simulink model "furnace_emul_v12"  (Simulink 5.0)
settings: Solver=FixedStepDiscrete  StartTime=0.0  StopTime=9000  RelTol=1e-3
values from neighbouring files (symbols this model uses):
  A_amb = pi*(D_e+2*d_ins)*L    (= 0.0498884492)    [tube_ini.m]
  A_e = pi*D_e*L    (= 0.0247557292)    [tube_ini.m]
  A_pi = pi*D_pi*L    (= 0.017592904)    [tube_ini.m]
  A_po = pi*D_po*L    (= 0.0184725492)    [tube_ini.m]
  A_w = pi/4*D_w^2*n_sl    (= 0.0628318)    [tube_ini.m]
  A_wc = pi*D_w*Li    (= 0.01256636)    [tube_ini.m]
  D_pi = D_w+2*DX_R    (= 0.28)    [tube_ini.m]
  D_w = 0.2    [tube_ini.m]
  elem_tmax = 1250    [tube_ini.m]
  F_A_e = lam_p_bct*F_A_e+lam_p_bcb*F_A_e([n:-1:1])    [tube_ini.m]
  F_A_ew = e_ew*A_ew./((1/ei-1)+(1/eo-1)*D_pi/D_w+1./(toeplitz(F1*Li)))    [tube_ini.m]
  F_A_p = lam_p_bct*F_A_p+lam_p_bcb*F_A_p([n:-1:1])    [tube_ini.m]
  F_A_pe = A_ep./((1/ei-1)+(1/eo-1)*D_po/D_e+1./(toeplitz(F1*Li)))    [tube_ini.m]
  F_A_pw = A_pw./((1/ei-1)+(1/eo-1)*D_pi/D_w+1./(toeplitz(F1*Li)))    [tube_ini.m]
  f_amb_ped = 1    [tube_ini.m]
  f_amb_top = .3    (= 0.3)    [tube_ini.m]
  Fb_A_ew = e_ew*Aib./((1/ei-1)+(1/eo-1)*Aib/A+1./(F4*Li))    [tube_ini.m]
  Fb_A_pw = Aib./((1/ei-1)+(1/eo-1)*Aib/A+1./(F4*Li))    [tube_ini.m]
  Fs_e = e_ew*A_e./((1/eo-1)+(1/eo-1)+1./(toeplitz(F5*Li)))    [tube_ini.m]
  Fs_p = A_pi./((1/eo-1)+(1/eo-1)+1./(toeplitz(F5*Li)))    [tube_ini.m]
  gww_bot = ones(N_w,1)*SW    [tube_ini.m]
  gww_top = gww_bot    [tube_ini.m]
  h_amb = 1    [tube_ini.m]
  h_gas = 2    [tube_ini.m]
  H_Z = zeros(n,5)    [tube_ini.m]
  k_adj_ped = 0.6    [tube_ini.m]
  k_adj_top = 0.5    [tube_ini.m]
  L = 0.2    [M_Hist040407.m]    (also in exp303.m = 500:499+ly; tube_ini.m = 0.02)
  lam_p_bcb = 1    [tube_ini.m]
  lam_p_bct = .4    (= 0.4)    [tube_ini.m]
  Li = dx_w    (= 0.02)    [tube_ini.m]
  m_e = rho_e*V_e    (= 0.6312710946)    [tube_ini.m]
  m_p = V_p*rho_p    (= 0.30294980688)    [tube_ini.m]
  m_ped = V_ped*rho_p    (= 1.5079632)    [tube_ini.m]
  m_top = rho_p*V_top    (= 1.5079632)    [tube_ini.m]
  m_w = rho_w*V_w    (= 0.146398094)    [tube_ini.m]
  mcp_adj_ped = 0.36    [tube_ini.m]
  mcp_adj_top = 0.25    [tube_ini.m]
  n = N_w+N_top+N_ped    [tube_ini.m]
  N_ped = round(DX_P/Li)    [tube_ini.m]
  N_top = n-N_w-N_p    [s_tubew.m]    (also in tube_ini.m = round(DX_T/Li))
  N_w = 100/n_sl    (= 50)    [tube_ini.m]
  pow_pm = pow_pml*pi*D_e*n*L/(d_e+d_g)    [tube_ini.m]
  pr_gas = 0.2    [tube_ini.m]
  PRG = 0*SPE; for ii=1:length(profile_loc); PRG(ii,profile_loc(ii))=1;end    [tube_ini.m]
  profile_loc = [N_top,h_zones(1)+round(h_zones(2)/2),   sum(h_zones(1:2))+round(h_zones(3)/2),sum(h_zones(1:3))+round(h_zones(4)/2),   n-N_ped]    [tube_ini.m]
  PRT = PRT'    [tube_ini.m]
  PRW = PRW'    [tube_ini.m]
  SPE = SPE'    [tube_ini.m]
  spike_loc = [round(h_zones(1)/2),h_zones(1)+round(h_zones(2)/2),   sum(h_zones(1:2))+round(h_zones(3)/2),sum(h_zones(1:3))+round(h_zones(4)/2),   sum(h_zones(1:4))+round(h_zones(5)/2)]    [tube_ini.m]
  SPT = SPT'    [tube_ini.m]
  T_0 = T_01*ones(n,1)    [tube_ini.m]
  T_a0 = T_a01*ones(n,1)    [tube_ini.m]
  T_amb = 25    [tube_ini.m]
  T_w0 = T_amb*ones(N_w,1)    [tube_ini.m]
  T_w0_ped = T_amb*ones(N_ped,1)    [tube_ini.m]
  T_w0_top = T_01*ones(N_top,1)    [tube_ini.m]
  Tsa = .5    (= 0.5)    [tube_ini.m]
  tube_tmax = 1200    [tube_ini.m]
  V_a = pi/4*D_pi^2*L    (= 0.00123150328)    [tube_ini.m]
undefined symbols (not defined in the file or in its folder): N, s_tubew
libraries: simulink3 x19, simulink x2
(part 1 of 2)
settings Model: LastModifiedBy="Kostas  Tsakalis"  BlockReductionOpt=off  BooleanDataType=off  RTWOptions="-aEnforceIntegerDowncast=1 -aExtMode=0 -aFoldNonRolledExpr=1 -aForceParamTrailComments=0 -aGenerateComments=1 -aIgnoreCustomStorageClasses=0 -aIncHierarchyInIds=0 -aInlineInvariantSignals=0 -aLocalBlockOutputs=1 -aLogVarNameModifier=\"rt_\" -aRTWVerbose=1 -aRollThreshold=5 -aShowEliminatedStatements=1"

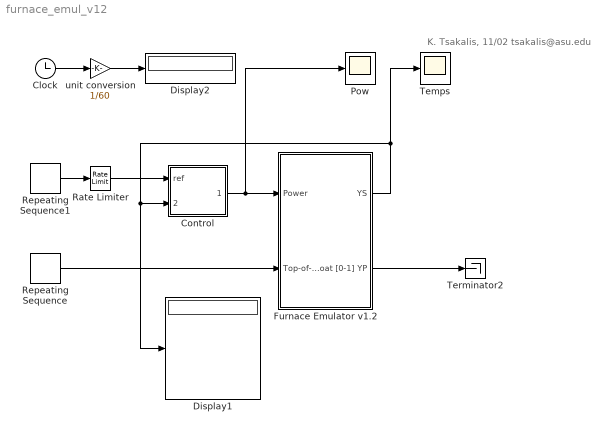
== system furnace_emul_v12 ==
  note: K. Tsakalis, 11/02
      | tsakalis@asu.edu
  Clock : Clock
      settings: Decimation=10
  Control : Subsystem
      mask init:
      | Tsa=0.5;
  Display1 : Display
      settings: Format=short_e
  Display2 : Display
      settings: Format=short_e
  Furnace Emulator v1.2 : Subsystem
      mask init:
      | tube_ini;
  Pow : Scope
      settings: TimeRange=6000  YMin=0  YMax=1
  Rate Limiter : RateLimiter  RisingSlewLimit=250/60  FallingSlewLimit=-200/60
  Repeating Sequence : simulink/Sources/Repeating Sequence  rep_seq_t="[0,  20,  22,  130,  132,  150]*60"  rep_seq_y="[1,  1,  0,  0,  1,  1]"
  Repeating Sequence1 : simulink/Sources/Repeating Sequence  rep_seq_t="[0,  35,  35.0001,  70,   70.0001  150 ]*60"  rep_seq_y="[0,  0,  300,  300,  0,  0]+600"
  Temps : Scope
      settings: TimeRange=6000  YMin=500  YMax=1000
  Terminator2 : Terminator
  unit conversion : Gain  Gain=1/60  SaturateOnIntegerOverflow=on
  wires:
  Furnace Emulator v1.2/1(YS) -> Temps/1, Control/2(meas), Display1/1
  Furnace Emulator v1.2/2(YP) -> Terminator2/1
  Clock/1 -> unit conversion/1
  Repeating Sequence1/1 -> Rate Limiter/1
  Control/1(Out1) -> Furnace Emulator v1.2/1(Power), Pow/1
  Rate Limiter/1 -> Control/1(ref)
  Repeating Sequence/1 -> Furnace Emulator v1.2/2(Top-of-boat [0-1])
  unit conversion/1 -> Display2/1

== system furnace_emul_v12/Control ==
  ref : Inport
  meas : Inport  Port=2
  "AW-PID " : Subsystem  mask(Anti-windup PID ){@1=[.005, 50, 10], @2=1, @3=0, @4=Tsa, @5=[1 0]}
      mask prompts: @1 "Gain kp - Integral time ki - Derivative time kd"; @2 "Pseudo-derivative filter time constant"; @3 "Error lowpass filter Time constant"; @4 "Sampling Time"; @5 "Saturation Limits [umax umin]"
      mask help: Discrete PID with Anti-windup and with lowpass filter
      mask init:
      | kp=@1(1);ki=@1(2);kd=@1(3);SAM=@2;TF=@3;DT=@4;umax=@5(1);umin=@5(2);
      mask Display: disp('AW-PID+filter')
  AW-PID 1 : Subsystem  mask(Anti-windup PID ){@1=[.005, 50, 10], @2=1, @3=0, @4=Tsa, @5=[1 0]}
      mask prompts: @1 "Gain kp - Integral time ki - Derivative time kd"; @2 "Pseudo-derivative filter time constant"; @3 "Error lowpass filter Time constant"; @4 "Sampling Time"; @5 "Saturation Limits [umax umin]"
      mask help: Discrete PID with Anti-windup and with lowpass filter
      mask init:
      | kp=@1(1);ki=@1(2);kd=@1(3);SAM=@2;TF=@3;DT=@4;umax=@5(1);umin=@5(2);
      mask Display: disp('AW-PID+filter')
  AW-PID 2 : Subsystem  mask(Anti-windup PID ){@1=[.005, 50, 10], @2=1, @3=0, @4=Tsa, @5=[1 0]}
      mask prompts: @1 "Gain kp - Integral time ki - Derivative time kd"; @2 "Pseudo-derivative filter time constant"; @3 "Error lowpass filter Time constant"; @4 "Sampling Time"; @5 "Saturation Limits [umax umin]"
      mask help: Discrete PID with Anti-windup and with lowpass filter
      mask init:
      | kp=@1(1);ki=@1(2);kd=@1(3);SAM=@2;TF=@3;DT=@4;umax=@5(1);umin=@5(2);
      mask Display: disp('AW-PID+filter')
  AW-PID 3 : Subsystem  mask(Anti-windup PID ){@1=[.005, 50, 10], @2=1, @3=0, @4=Tsa, @5=[1 0]}
      mask prompts: @1 "Gain kp - Integral time ki - Derivative time kd"; @2 "Pseudo-derivative filter time constant"; @3 "Error lowpass filter Time constant"; @4 "Sampling Time"; @5 "Saturation Limits [umax umin]"
      mask help: Discrete PID with Anti-windup and with lowpass filter
      mask init:
      | kp=@1(1);ki=@1(2);kd=@1(3);SAM=@2;TF=@3;DT=@4;umax=@5(1);umin=@5(2);
      mask Display: disp('AW-PID+filter')
  AW-PID 4 : Subsystem  mask(Anti-windup PID ){@1=[.005, 50, 10], @2=1, @3=0, @4=Tsa, @5=[1 0]}
      mask prompts: @1 "Gain kp - Integral time ki - Derivative time kd"; @2 "Pseudo-derivative filter time constant"; @3 "Error lowpass filter Time constant"; @4 "Sampling Time"; @5 "Saturation Limits [umax umin]"
      mask help: Discrete PID with Anti-windup and with lowpass filter
      mask init:
      | kp=@1(1);ki=@1(2);kd=@1(3);SAM=@2;TF=@3;DT=@4;umax=@5(1);umin=@5(2);
      mask Display: disp('AW-PID+filter')
  Mux1 : Mux  Inputs=5
  Selector1 : Selector  Elements=2  InputPortWidth=5
  Selector2 : Selector  Elements=3  InputPortWidth=5
  Selector3 : Selector  Elements=4  InputPortWidth=5
  Selector4 : Selector  Elements=5  InputPortWidth=5
  Selector5 : Selector  InputPortWidth=5
  Out1 : Outport
  wires:
  ref/1 -> "AW-PID "/1(Set point), AW-PID 1/1(Set point), AW-PID 2/1(Set point), AW-PID 3/1(Set point), AW-PID 4/1(Set point)
  Mux1/1 -> Out1/1
  meas/1 -> Selector5/1, Selector1/1, Selector2/1, Selector3/1, Selector4/1
  Selector5/1 -> "AW-PID "/2(System Output)
  Selector4/1 -> AW-PID 4/2(System Output)
  Selector3/1 -> AW-PID 3/2(System Output)
  Selector2/1 -> AW-PID 2/2(System Output)
  Selector1/1 -> AW-PID 1/2(System Output)
  AW-PID 2/1(Input to system) -> Mux1/3
  "AW-PID "/1(Input to system) -> Mux1/1
  AW-PID 1/1(Input to system) -> Mux1/2
  AW-PID 3/1(Input to system) -> Mux1/4
  AW-PID 4/1(Input to system) -> Mux1/5

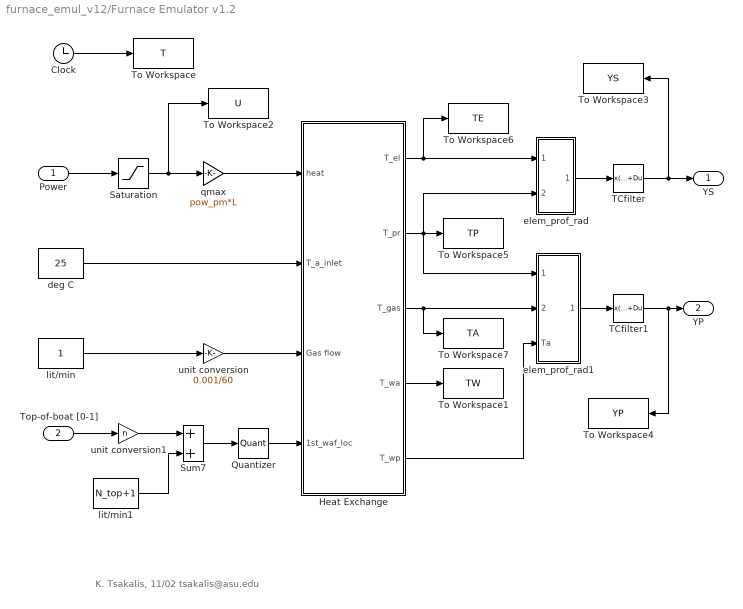
== system furnace_emul_v12/Furnace Emulator v1.2 ==
  note: K. Tsakalis, 11/02
      | tsakalis@asu.edu
  Power : Inport
  Top-of-boat [0-1] : Inport  Port=2
  Clock : Clock
      settings: Decimation=10
  Heat Exchange : Subsystem
  Quantizer : Quantizer  QuantizationInterval=1
  Saturation : Saturate  UpperLimit=1  LowerLimit=0
  Sum7 : Sum  Inputs=2  SaturateOnIntegerOverflow=on  InputSameDT=on
  TCfilter : DiscreteStateSpace  A=eye(5,5)-eye(5,5)*0.1*Tsa  B=eye(5,5)*0.1*Tsa  C=eye(5,5)  D=zeros(5,5)  X0=T_0(spike_loc)  SampleTime=Tsa
  TCfilter1 : DiscreteStateSpace  A=eye(5,5)-eye(5,5)*0.1*Tsa  B=eye(5,5)*0.1*Tsa  C=eye(5,5)  D=zeros(5,5)  X0=(T_0(profile_loc)*0.8+T_a0(profile_loc)*0.2)  SampleTime=Tsa
  To Workspace : ToWorkspace  VariableName=T  SampleTime=Tsa  SaveFormat=Array
      settings: Decimation=decim
  To Workspace1 : ToWorkspace  VariableName=TW  SampleTime=Tsa  SaveFormat=Array
      settings: Decimation=decim
  To Workspace2 : ToWorkspace  VariableName=U  SampleTime=Tsa  SaveFormat=Array
      settings: Decimation=decim
  To Workspace3 : ToWorkspace  VariableName=YS  SampleTime=Tsa  SaveFormat=Array
      settings: Decimation=decim
  To Workspace4 : ToWorkspace  VariableName=YP  SampleTime=Tsa  SaveFormat=Array
      settings: Decimation=decim
  To Workspace5 : ToWorkspace  VariableName=TP  SampleTime=Tsa  SaveFormat=Array
      settings: Decimation=decim
  To Workspace6 : ToWorkspace  VariableName=TE  SampleTime=Tsa  SaveFormat=Array
      settings: Decimation=decim
  To Workspace7 : ToWorkspace  VariableName=TA  SampleTime=Tsa  SaveFormat=Array
      settings: Decimation=decim
  deg C : Constant  Value=25
  elem_prof_rad : Subsystem
  elem_prof_rad1 : Subsystem
  lit/min : Constant
  lit/min1 : Constant  Value=N_top+1
  qmax : Gain  Gain=pow_pm*L  SaturateOnIntegerOverflow=on
  unit conversion : Gain  Gain=0.001/60  SaturateOnIntegerOverflow=on
  unit conversion1 : Gain  Gain=n  SaturateOnIntegerOverflow=on
  YS : Outport
  YP : Outport  Port=2
  wires:
  unit conversion/1 -> Heat Exchange/3(Gas flow)
  Power/1 -> Saturation/1
  Saturation/1 -> qmax/1, To Workspace2/1
  deg C/1 -> Heat Exchange/2(T_a_inlet)
  qmax/1 -> Heat Exchange/1(heat)
  Heat Exchange/1(T_el) -> To Workspace6/1, elem_prof_rad/1(Tel)
  Heat Exchange/2(T_pr) -> To Workspace5/1, elem_prof_rad/2(Ttu), elem_prof_rad1/1(Ttu)
  Heat Exchange/4(T_wa) -> To Workspace1/1
  Heat Exchange/3(T_gas) -> To Workspace7/1, elem_prof_rad1/2(Twa)
  elem_prof_rad/1(Tav) -> TCfilter/1
  elem_prof_rad1/1(Tav) -> TCfilter1/1
  TCfilter/1 -> YS/1, To Workspace3/1
  TCfilter1/1 -> YP/1, To Workspace4/1
  Clock/1 -> To Workspace/1
  Heat Exchange/5(T_wp) -> elem_prof_rad1/3(Ta)
  Top-of-boat [0-1]/1 -> unit conversion1/1
  lit/min/1 -> unit conversion/1
  Quantizer/1 -> Heat Exchange/4(1st_waf_loc)
  Sum7/1 -> Quantizer/1
  unit conversion1/1 -> Sum7/1
  lit/min1/1 -> Sum7/2

== system furnace_emul_v12/Control/AW-PID  ==
  Set point : Inport
  System Output : Inport  Port=2
  Constant : Constant  Value=0
  Dis. Transfer Fcn1 : DiscreteTransferFcn  Numerator=[DT/SAM]  Denominator=[1 -1+DT/SAM]  SampleTime=DT
  Low-pass filter : DiscreteTransferFcn  Numerator="[DT/(TF+DT),  0]"  Denominator="[1,  -TF/(TF+DT)]"  SampleTime=DT
  P+I+D : Sum  Inputs=++++-  SaturateOnIntegerOverflow=on  InputSameDT=on
  Proportional : Gain  Gain=kp  SaturateOnIntegerOverflow=on
  Proportional3 : Gain  Gain=kp*kd/SAM  SaturateOnIntegerOverflow=on
  Saturation : Saturate  UpperLimit=umax  LowerLimit=umin
  error : Sum  Inputs=+-  SaturateOnIntegerOverflow=on  InputSameDT=on
  gain : Gain  Gain=DT*kp/ki  SaturateOnIntegerOverflow=on
  integrator2 : Subsystem  mask(Anti windup intgrator){@1=umax, @2=umin, @3=DT}
      mask prompts: @1 "umax"; @2 "umin"; @3 "sampling time"
      mask help: Integral with anti-windup
      mask init:
      | umax=@1 ; umin =@2 ;DT=@3;
      mask Display: disp('DT-I-AW')
  Input to system : Outport  InitialOutput=0
  wires:
  integrator2/1(out_1) -> P+I+D/1
  error/1 -> Low-pass filter/1
  Set point/1 -> error/1
  System Output/1 -> error/2
  Proportional3/1 -> Dis. Transfer Fcn1/1, P+I+D/4
  Low-pass filter/1 -> Proportional/1, Proportional3/1, gain/1
  Dis. Transfer Fcn1/1 -> P+I+D/5
  Proportional/1 -> P+I+D/3
  gain/1 -> integrator2/1(in_1)
  P+I+D/1 -> Saturation/1
  Saturation/1 -> Input to system/1
  Constant/1 -> P+I+D/2

== system furnace_emul_v12/Control/AW-PID 1 ==
  Set point : Inport
  System Output : Inport  Port=2
  Constant : Constant  Value=0
  Dis. Transfer Fcn1 : DiscreteTransferFcn  Numerator=[DT/SAM]  Denominator=[1 -1+DT/SAM]  SampleTime=DT
  Low-pass filter : DiscreteTransferFcn  Numerator="[DT/(TF+DT),  0]"  Denominator="[1,  -TF/(TF+DT)]"  SampleTime=DT
  P+I+D : Sum  Inputs=++++-  SaturateOnIntegerOverflow=on  InputSameDT=on
  Proportional : Gain  Gain=kp  SaturateOnIntegerOverflow=on
  Proportional3 : Gain  Gain=kp*kd/SAM  SaturateOnIntegerOverflow=on
  Saturation : Saturate  UpperLimit=umax  LowerLimit=umin
  error : Sum  Inputs=+-  SaturateOnIntegerOverflow=on  InputSameDT=on
  gain : Gain  Gain=DT*kp/ki  SaturateOnIntegerOverflow=on
  integrator2 : Subsystem  mask(Anti windup intgrator){@1=umax, @2=umin, @3=DT}
      mask prompts: @1 "umax"; @2 "umin"; @3 "sampling time"
      mask help: Integral with anti-windup
      mask init:
      | umax=@1 ; umin =@2 ;DT=@3;
      mask Display: disp('DT-I-AW')
  Input to system : Outport  InitialOutput=0
  wires:
  Constant/1 -> P+I+D/2
  Saturation/1 -> Input to system/1
  P+I+D/1 -> Saturation/1
  gain/1 -> integrator2/1(in_1)
  Proportional/1 -> P+I+D/3
  Dis. Transfer Fcn1/1 -> P+I+D/5
  Low-pass filter/1 -> gain/1, Proportional3/1, Proportional/1
  Proportional3/1 -> P+I+D/4, Dis. Transfer Fcn1/1
  System Output/1 -> error/2
  Set point/1 -> error/1
  error/1 -> Low-pass filter/1
  integrator2/1(out_1) -> P+I+D/1

== system furnace_emul_v12/Control/AW-PID 2 ==
  Set point : Inport
  System Output : Inport  Port=2
  Constant : Constant  Value=0
  Dis. Transfer Fcn1 : DiscreteTransferFcn  Numerator=[DT/SAM]  Denominator=[1 -1+DT/SAM]  SampleTime=DT
  Low-pass filter : DiscreteTransferFcn  Numerator="[DT/(TF+DT),  0]"  Denominator="[1,  -TF/(TF+DT)]"  SampleTime=DT
  P+I+D : Sum  Inputs=++++-  SaturateOnIntegerOverflow=on  InputSameDT=on
  Proportional : Gain  Gain=kp  SaturateOnIntegerOverflow=on
  Proportional3 : Gain  Gain=kp*kd/SAM  SaturateOnIntegerOverflow=on
  Saturation : Saturate  UpperLimit=umax  LowerLimit=umin
  error : Sum  Inputs=+-  SaturateOnIntegerOverflow=on  InputSameDT=on
  gain : Gain  Gain=DT*kp/ki  SaturateOnIntegerOverflow=on
  integrator2 : Subsystem  mask(Anti windup intgrator){@1=umax, @2=umin, @3=DT}
      mask prompts: @1 "umax"; @2 "umin"; @3 "sampling time"
      mask help: Integral with anti-windup
      mask init:
      | umax=@1 ; umin =@2 ;DT=@3;
      mask Display: disp('DT-I-AW')
  Input to system : Outport  InitialOutput=0
  wires:
  integrator2/1(out_1) -> P+I+D/1
  error/1 -> Low-pass filter/1
  Set point/1 -> error/1
  System Output/1 -> error/2
  Proportional3/1 -> Dis. Transfer Fcn1/1, P+I+D/4
  Low-pass filter/1 -> Proportional/1, Proportional3/1, gain/1
  Dis. Transfer Fcn1/1 -> P+I+D/5
  Proportional/1 -> P+I+D/3
  gain/1 -> integrator2/1(in_1)
  P+I+D/1 -> Saturation/1
  Saturation/1 -> Input to system/1
  Constant/1 -> P+I+D/2

== system furnace_emul_v12/Control/AW-PID 3 ==
  Set point : Inport
  System Output : Inport  Port=2
  Constant : Constant  Value=0
  Dis. Transfer Fcn1 : DiscreteTransferFcn  Numerator=[DT/SAM]  Denominator=[1 -1+DT/SAM]  SampleTime=DT
  Low-pass filter : DiscreteTransferFcn  Numerator="[DT/(TF+DT),  0]"  Denominator="[1,  -TF/(TF+DT)]"  SampleTime=DT
  P+I+D : Sum  Inputs=++++-  SaturateOnIntegerOverflow=on  InputSameDT=on
  Proportional : Gain  Gain=kp  SaturateOnIntegerOverflow=on
  Proportional3 : Gain  Gain=kp*kd/SAM  SaturateOnIntegerOverflow=on
  Saturation : Saturate  UpperLimit=umax  LowerLimit=umin
  error : Sum  Inputs=+-  SaturateOnIntegerOverflow=on  InputSameDT=on
  gain : Gain  Gain=DT*kp/ki  SaturateOnIntegerOverflow=on
  integrator2 : Subsystem  mask(Anti windup intgrator){@1=umax, @2=umin, @3=DT}
      mask prompts: @1 "umax"; @2 "umin"; @3 "sampling time"
      mask help: Integral with anti-windup
      mask init:
      | umax=@1 ; umin =@2 ;DT=@3;
      mask Display: disp('DT-I-AW')
  Input to system : Outport  InitialOutput=0
  wires:
  Constant/1 -> P+I+D/2
  Saturation/1 -> Input to system/1
  P+I+D/1 -> Saturation/1
  gain/1 -> integrator2/1(in_1)
  Proportional/1 -> P+I+D/3
  Dis. Transfer Fcn1/1 -> P+I+D/5
  Low-pass filter/1 -> gain/1, Proportional3/1, Proportional/1
  Proportional3/1 -> P+I+D/4, Dis. Transfer Fcn1/1
  System Output/1 -> error/2
  Set point/1 -> error/1
  error/1 -> Low-pass filter/1
  integrator2/1(out_1) -> P+I+D/1

== system furnace_emul_v12/Control/AW-PID 4 ==
  Set point : Inport
  System Output : Inport  Port=2
  Constant : Constant  Value=0
  Dis. Transfer Fcn1 : DiscreteTransferFcn  Numerator=[DT/SAM]  Denominator=[1 -1+DT/SAM]  SampleTime=DT
  Low-pass filter : DiscreteTransferFcn  Numerator="[DT/(TF+DT),  0]"  Denominator="[1,  -TF/(TF+DT)]"  SampleTime=DT
  P+I+D : Sum  Inputs=++++-  SaturateOnIntegerOverflow=on  InputSameDT=on
  Proportional : Gain  Gain=kp  SaturateOnIntegerOverflow=on
  Proportional3 : Gain  Gain=kp*kd/SAM  SaturateOnIntegerOverflow=on
  Saturation : Saturate  UpperLimit=umax  LowerLimit=umin
  error : Sum  Inputs=+-  SaturateOnIntegerOverflow=on  InputSameDT=on
  gain : Gain  Gain=DT*kp/ki  SaturateOnIntegerOverflow=on
  integrator2 : Subsystem  mask(Anti windup intgrator){@1=umax, @2=umin, @3=DT}
      mask prompts: @1 "umax"; @2 "umin"; @3 "sampling time"
      mask help: Integral with anti-windup
      mask init:
      | umax=@1 ; umin =@2 ;DT=@3;
      mask Display: disp('DT-I-AW')
  Input to system : Outport  InitialOutput=0
  wires:
  integrator2/1(out_1) -> P+I+D/1
  error/1 -> Low-pass filter/1
  Set point/1 -> error/1
  System Output/1 -> error/2
  Proportional3/1 -> Dis. Transfer Fcn1/1, P+I+D/4
  Low-pass filter/1 -> Proportional/1, Proportional3/1, gain/1
  Dis. Transfer Fcn1/1 -> P+I+D/5
  Proportional/1 -> P+I+D/3
  gain/1 -> integrator2/1(in_1)
  P+I+D/1 -> Saturation/1
  Saturation/1 -> Input to system/1
  Constant/1 -> P+I+D/2

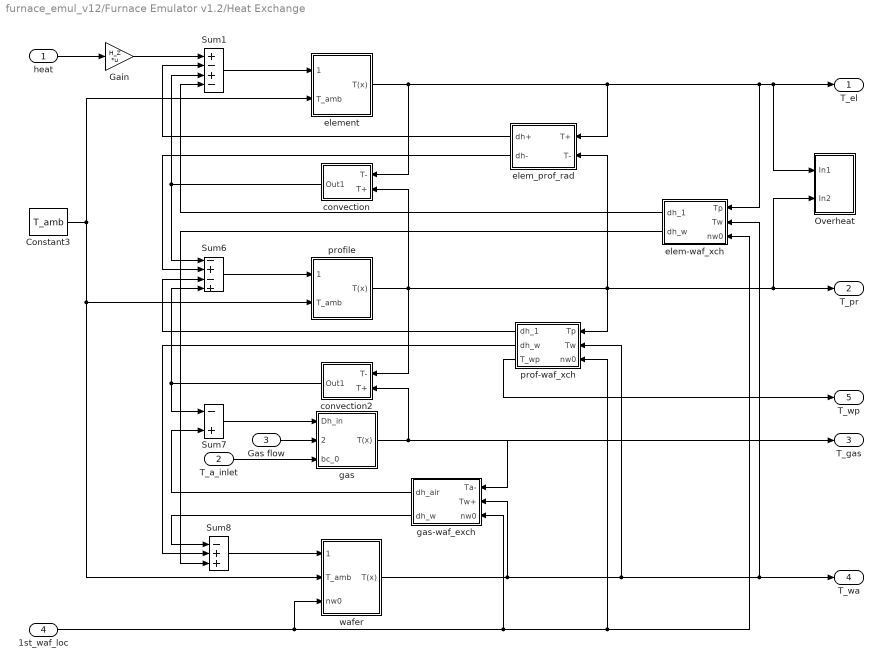
== system furnace_emul_v12/Furnace Emulator v1.2/Heat Exchange ==
  heat : Inport
  T_a_inlet : Inport  Port=2
  Gas flow : Inport  Port=3
  1st_waf_loc : Inport  Port=4
  Constant3 : Constant  Value=T_amb
  Gain : Gain  Gain=H_Z  Multiplication=Matrix(K*u)  SaturateOnIntegerOverflow=on
  Overheat : Subsystem
  Sum1 : Sum  Inputs=+-+-  SaturateOnIntegerOverflow=on  InputSameDT=on
  Sum6 : Sum  Inputs=-+-+  SaturateOnIntegerOverflow=on  InputSameDT=on
  Sum7 : Sum  Inputs=-+  SaturateOnIntegerOverflow=on  InputSameDT=on
  Sum8 : Sum  Inputs=-++  SaturateOnIntegerOverflow=on  InputSameDT=on
  convection : Subsystem  Orientation=left
  convection2 : Subsystem  Orientation=left
  elem-waf_xch : Subsystem  Orientation=left
  elem_prof_rad : Subsystem  Orientation=left
  element : Subsystem
  gas : Subsystem
  gas-waf_exch : Subsystem  Orientation=left
  prof-waf_xch : Subsystem  Orientation=left
  profile : Subsystem
  wafer : Subsystem
  T_el : Outport
  T_pr : Outport  Port=2
  T_gas : Outport  Port=3
  T_wa : Outport  Port=4
  T_wp : Outport  Port=5
  wires:
  T_a_inlet/1 -> gas/3(bc_0)
  Gas flow/1 -> gas/2(gas flow)
  gas/1(T(x)) -> gas-waf_exch/1(Ta-), convection2/2(T+), T_gas/1
  heat/1 -> Gain/1
  Sum1/1 -> element/1(heat_in)
  element/1(T(x)) -> elem_prof_rad/1(T+), elem-waf_xch/1(Tp), T_el/1, Overheat/1(In1), convection/1(T-)
  convection/1(Out1) -> Sum6/1, Sum1/3
  Constant3/1 -> element/2(T_amb), profile/2(T_amb), wafer/2(T_amb)
  profile/1(T(x)) -> convection2/1(T-), elem_prof_rad/2(T-), prof-waf_xch/1(Tp), T_pr/1, Overheat/2(In2), convection/2(T+)
  Sum6/1 -> profile/1(heat_in)
  Sum7/1 -> gas/1(Dh_in)
  convection2/1(Out1) -> Sum7/1, Sum6/4
  wafer/1(T(x)) -> prof-waf_xch/2(Tw), T_wa/1, elem-waf_xch/2(Tw), gas-waf_exch/2(Tw+)
  Sum8/1 -> wafer/1(heat_in)
  gas-waf_exch/2(dh_w) -> Sum8/1
  gas-waf_exch/1(dh_air) -> Sum7/2
  1st_waf_loc/1 -> wafer/3(nw0), gas-waf_exch/3(nw0), prof-waf_xch/3(nw0), elem-waf_xch/3(nw0)
  elem_prof_rad/2(dh-) -> Sum6/2
  prof-waf_xch/2(dh_w) -> Sum8/2
  prof-waf_xch/1(dh_1) -> Sum6/3
  elem_prof_rad/1(dh+) -> Sum1/2
  Gain/1 -> Sum1/1
  prof-waf_xch/3(T_wp) -> T_wp/1
  elem-waf_xch/1(dh_1) -> Sum1/4
  elem-waf_xch/2(dh_w) -> Sum8/3

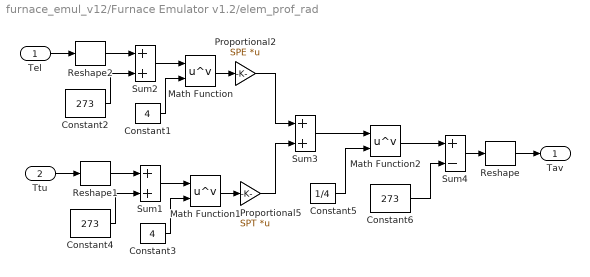
== system furnace_emul_v12/Furnace Emulator v1.2/elem_prof_rad ==
  Tel : Inport
  Ttu : Inport  Port=2
  Constant1 : Constant  Value=4
  Constant2 : Constant  Value=273
  Constant3 : Constant  Value=4
  Constant4 : Constant  Value=273
  Constant5 : Constant  Value=1/4
  Constant6 : Constant  Value=273
  Math Function : Math  Operator=pow
  Math Function1 : Math  Operator=pow
  Math Function2 : Math  Operator=pow
  Proportional2 : Gain  Gain=SPE  Multiplication=Matrix(K*u)  SaturateOnIntegerOverflow=on
  Proportional5 : Gain  Gain=SPT  Multiplication=Matrix(K*u)  SaturateOnIntegerOverflow=on
  Reshape : simulink3/Signals & Systems/Reshape  OutputDimensionality=1-D array  OutputDimensions=[1,1]
  Reshape1 : simulink3/Signals & Systems/Reshape  OutputDimensionality=Column vector  OutputDimensions=[1,1]
  Reshape2 : simulink3/Signals & Systems/Reshape  OutputDimensionality=Column vector  OutputDimensions=[1,1]
  Sum1 : Sum  Inputs=2  SaturateOnIntegerOverflow=on  InputSameDT=on
  Sum2 : Sum  Inputs=2  SaturateOnIntegerOverflow=on  InputSameDT=on
  Sum3 : Sum  SaturateOnIntegerOverflow=on  InputSameDT=on
  Sum4 : Sum  Inputs=+-  SaturateOnIntegerOverflow=on  InputSameDT=on
  Tav : Outport
  wires:
  Constant6/1 -> Sum4/2
  Sum4/1 -> Reshape/1
  Math Function2/1 -> Sum4/1
  Constant5/1 -> Math Function2/2
  Sum3/1 -> Math Function2/1
  Proportional5/1 -> Sum3/2
  Proportional2/1 -> Sum3/1
  Constant1/1 -> Math Function/2
  Sum2/1 -> Math Function/1
  Constant2/1 -> Sum2/2
  Tel/1 -> Reshape2/1
  Constant3/1 -> Math Function1/2
  Sum1/1 -> Math Function1/1
  Constant4/1 -> Sum1/2
  Ttu/1 -> Reshape1/1
  Math Function/1 -> Proportional2/1
  Math Function1/1 -> Proportional5/1
  Reshape/1 -> Tav/1
  Reshape1/1 -> Sum1/1
  Reshape2/1 -> Sum2/1

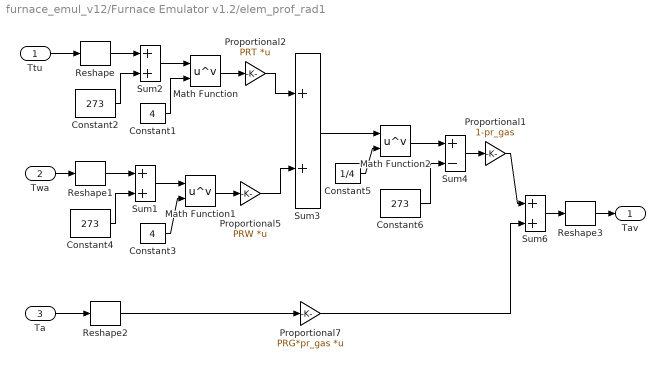
== system furnace_emul_v12/Furnace Emulator v1.2/elem_prof_rad1 ==
  Ttu : Inport
  Twa : Inport  Port=2
  Ta : Inport  Port=3
  Constant1 : Constant  Value=4
  Constant2 : Constant  Value=273
  Constant3 : Constant  Value=4
  Constant4 : Constant  Value=273
  Constant5 : Constant  Value=1/4
  Constant6 : Constant  Value=273
  Math Function : Math  Operator=pow
  Math Function1 : Math  Operator=pow
  Math Function2 : Math  Operator=pow
  Proportional1 : Gain  Gain=1-pr_gas  SaturateOnIntegerOverflow=on
  Proportional2 : Gain  Gain=PRT  Multiplication=Matrix(K*u)  SaturateOnIntegerOverflow=on
  Proportional5 : Gain  Gain=PRW  Multiplication=Matrix(K*u)  SaturateOnIntegerOverflow=on
  Proportional7 : Gain  Gain=PRG*pr_gas  Multiplication=Matrix(K*u)  SaturateOnIntegerOverflow=on
  Reshape : simulink3/Signals & Systems/Reshape  OutputDimensionality=Column vector  OutputDimensions=[1,1]
  Reshape1 : simulink3/Signals & Systems/Reshape  OutputDimensionality=Column vector  OutputDimensions=[1,1]
  Reshape2 : simulink3/Signals & Systems/Reshape  OutputDimensionality=Column vector  OutputDimensions=[1,1]
  Reshape3 : simulink3/Signals & Systems/Reshape  OutputDimensionality=1-D array  OutputDimensions=[1,1]
  Sum1 : Sum  Inputs=2  SaturateOnIntegerOverflow=on  InputSameDT=on
  Sum2 : Sum  Inputs=2  SaturateOnIntegerOverflow=on  InputSameDT=on
  Sum3 : Sum  SaturateOnIntegerOverflow=on  InputSameDT=on
  Sum4 : Sum  Inputs=+-  SaturateOnIntegerOverflow=on  InputSameDT=on
  Sum6 : Sum  Inputs=2  SaturateOnIntegerOverflow=on  InputSameDT=on
  Tav : Outport
  wires:
  Math Function1/1 -> Proportional5/1
  Math Function/1 -> Proportional2/1
  Twa/1 -> Reshape1/1
  Constant4/1 -> Sum1/2
  Sum1/1 -> Math Function1/1
  Constant3/1 -> Math Function1/2
  Ttu/1 -> Reshape/1
  Constant2/1 -> Sum2/2
  Sum2/1 -> Math Function/1
  Constant1/1 -> Math Function/2
  Proportional2/1 -> Sum3/1
  Proportional5/1 -> Sum3/2
  Sum3/1 -> Math Function2/1
  Constant5/1 -> Math Function2/2
  Math Function2/1 -> Sum4/1
  Constant6/1 -> Sum4/2
  Ta/1 -> Reshape2/1
  Proportional7/1 -> Sum6/2
  Sum6/1 -> Reshape3/1
  Sum4/1 -> Proportional1/1
  Proportional1/1 -> Sum6/1
  Reshape/1 -> Sum2/1
  Reshape1/1 -> Sum1/1
  Reshape2/1 -> Proportional7/1
  Reshape3/1 -> Tav/1

== system furnace_emul_v12/Control/AW-PID /integrator2 ==
  in_1 : Inport
  Constant : Constant  Value=umax
  Constant3 : Constant  Value=umin
  Switch : Switch  SaturateOnIntegerOverflow=on  InputSameDT=on
  Switch2 : Switch  SaturateOnIntegerOverflow=on  InputSameDT=on
  delay : DiscreteTransferFcn  Orientation=left  Denominator=[1 0]  SampleTime=DT
  error1 : Sum  SaturateOnIntegerOverflow=on  InputSameDT=on
  error2 : Sum  Inputs=+-  SaturateOnIntegerOverflow=on  InputSameDT=on
  error3 : Sum  Inputs=+-  SaturateOnIntegerOverflow=on  InputSameDT=on
  out_1 : Outport  InitialOutput=0
  wires:
  delay/1 -> error1/1
  error2/1 -> Switch/2
  Constant/1 -> error2/1, Switch/3
  error1/1 -> error2/2, Switch/1
  error3/1 -> Switch2/2
  Constant3/1 -> error3/2, Switch2/3
  Switch/1 -> error3/1, Switch2/1
  Switch2/1 -> delay/1, out_1/1
  in_1/1 -> error1/2

== system furnace_emul_v12/Control/AW-PID 1/integrator2 ==
  in_1 : Inport
  Constant : Constant  Value=umax
  Constant3 : Constant  Value=umin
  Switch : Switch  SaturateOnIntegerOverflow=on  InputSameDT=on
  Switch2 : Switch  SaturateOnIntegerOverflow=on  InputSameDT=on
  delay : DiscreteTransferFcn  Orientation=left  Denominator=[1 0]  SampleTime=DT
  error1 : Sum  SaturateOnIntegerOverflow=on  InputSameDT=on
  error2 : Sum  Inputs=+-  SaturateOnIntegerOverflow=on  InputSameDT=on
  error3 : Sum  Inputs=+-  SaturateOnIntegerOverflow=on  InputSameDT=on
  out_1 : Outport  InitialOutput=0
  wires:
  in_1/1 -> error1/2
  Switch2/1 -> out_1/1, delay/1
  Switch/1 -> Switch2/1, error3/1
  Constant3/1 -> Switch2/3, error3/2
  error3/1 -> Switch2/2
  error1/1 -> Switch/1, error2/2
  Constant/1 -> Switch/3, error2/1
  error2/1 -> Switch/2
  delay/1 -> error1/1

== system furnace_emul_v12/Control/AW-PID 2/integrator2 ==
  in_1 : Inport
  Constant : Constant  Value=umax
  Constant3 : Constant  Value=umin
  Switch : Switch  SaturateOnIntegerOverflow=on  InputSameDT=on
  Switch2 : Switch  SaturateOnIntegerOverflow=on  InputSameDT=on
  delay : DiscreteTransferFcn  Orientation=left  Denominator=[1 0]  SampleTime=DT
  error1 : Sum  SaturateOnIntegerOverflow=on  InputSameDT=on
  error2 : Sum  Inputs=+-  SaturateOnIntegerOverflow=on  InputSameDT=on
  error3 : Sum  Inputs=+-  SaturateOnIntegerOverflow=on  InputSameDT=on
  out_1 : Outport  InitialOutput=0
  wires:
  delay/1 -> error1/1
  error2/1 -> Switch/2
  Constant/1 -> error2/1, Switch/3
  error1/1 -> error2/2, Switch/1
  error3/1 -> Switch2/2
  Constant3/1 -> error3/2, Switch2/3
  Switch/1 -> error3/1, Switch2/1
  Switch2/1 -> delay/1, out_1/1
  in_1/1 -> error1/2

== system furnace_emul_v12/Control/AW-PID 3/integrator2 ==
  in_1 : Inport
  Constant : Constant  Value=umax
  Constant3 : Constant  Value=umin
  Switch : Switch  SaturateOnIntegerOverflow=on  InputSameDT=on
  Switch2 : Switch  SaturateOnIntegerOverflow=on  InputSameDT=on
  delay : DiscreteTransferFcn  Orientation=left  Denominator=[1 0]  SampleTime=DT
  error1 : Sum  SaturateOnIntegerOverflow=on  InputSameDT=on
  error2 : Sum  Inputs=+-  SaturateOnIntegerOverflow=on  InputSameDT=on
  error3 : Sum  Inputs=+-  SaturateOnIntegerOverflow=on  InputSameDT=on
  out_1 : Outport  InitialOutput=0
  wires:
  in_1/1 -> error1/2
  Switch2/1 -> out_1/1, delay/1
  Switch/1 -> Switch2/1, error3/1
  Constant3/1 -> Switch2/3, error3/2
  error3/1 -> Switch2/2
  error1/1 -> Switch/1, error2/2
  Constant/1 -> Switch/3, error2/1
  error2/1 -> Switch/2
  delay/1 -> error1/1

== system furnace_emul_v12/Control/AW-PID 4/integrator2 ==
  in_1 : Inport
  Constant : Constant  Value=umax
  Constant3 : Constant  Value=umin
  Switch : Switch  SaturateOnIntegerOverflow=on  InputSameDT=on
  Switch2 : Switch  SaturateOnIntegerOverflow=on  InputSameDT=on
  delay : DiscreteTransferFcn  Orientation=left  Denominator=[1 0]  SampleTime=DT
  error1 : Sum  SaturateOnIntegerOverflow=on  InputSameDT=on
  error2 : Sum  Inputs=+-  SaturateOnIntegerOverflow=on  InputSameDT=on
  error3 : Sum  Inputs=+-  SaturateOnIntegerOverflow=on  InputSameDT=on
  out_1 : Outport  InitialOutput=0
  wires:
  delay/1 -> error1/1
  error2/1 -> Switch/2
  Constant/1 -> error2/1, Switch/3
  error1/1 -> error2/2, Switch/1
  error3/1 -> Switch2/2
  Constant3/1 -> error3/2, Switch2/3
  Switch/1 -> error3/1, Switch2/1
  Switch2/1 -> delay/1, out_1/1
  in_1/1 -> error1/2

== system furnace_emul_v12/Furnace Emulator v1.2/Heat Exchange/Overheat ==
  In1 : Inport
  In2 : Inport  Port=2
  Constant1 : Constant  Value=elem_tmax
  Constant2 : Constant  Value=tube_tmax
  Logical Operator : Logic  Operator=OR
  MinMax : MinMax  Function=max
  MinMax1 : MinMax  Function=max
  Relational Operator : RelationalOperator  Operator=>  InputSameDT=on
  Relational Operator1 : RelationalOperator  Operator=>  InputSameDT=on
  Stop Simulation : Stop
  wires:
  MinMax/1 -> Relational Operator/1
  Constant1/1 -> Relational Operator/2
  In1/1 -> MinMax/1
  In2/1 -> MinMax1/1
  MinMax1/1 -> Relational Operator1/1
  Relational Operator/1 -> Logical Operator/1
  Relational Operator1/1 -> Logical Operator/2
  Logical Operator/1 -> Stop Simulation/1
  Constant2/1 -> Relational Operator1/2

== system furnace_emul_v12/Furnace Emulator v1.2/Heat Exchange/convection ==
  T- : Inport  Orientation=left
  T+ : Inport  Orientation=left  Port=2
  Abs : Abs  Orientation=left  SaturateOnIntegerOverflow=on
  Constant3 : Constant  Value=0.25
  Math Function : Math  Orientation=left  Operator=pow
  Product : Product  Orientation=left  SaturateOnIntegerOverflow=on  InputSameDT=on
  Proportional2 : Gain  Orientation=left  Gain=1.42*A_e*A_po/(A_e+A_po)  SaturateOnIntegerOverflow=on
  Sum3 : Sum  Orientation=left  Inputs=-+  SaturateOnIntegerOverflow=on  InputSameDT=on
  Out1 : Outport  Orientation=left
  wires:
  Sum3/1 -> Abs/1, Product/1
  T-/1 -> Sum3/1
  T+/1 -> Sum3/2
  Abs/1 -> Math Function/1
  Constant3/1 -> Math Function/2
  Math Function/1 -> Proportional2/1
  Product/1 -> Out1/1
  Proportional2/1 -> Product/2

== system furnace_emul_v12/Furnace Emulator v1.2/Heat Exchange/convection2 ==
  T- : Inport  Orientation=left
  T+ : Inport  Orientation=left  Port=2
  Abs : Abs  Orientation=left  SaturateOnIntegerOverflow=on
  Constant3 : Constant  Value=0.25
  Math Function : Math  Orientation=left  Operator=pow
  Product : Product  Orientation=left  SaturateOnIntegerOverflow=on  InputSameDT=on
  Proportional2 : Gain  Orientation=left  Gain=1.42*A_pi*h_gas  SaturateOnIntegerOverflow=on
  Sum3 : Sum  Orientation=left  Inputs=-+  SaturateOnIntegerOverflow=on  InputSameDT=on
  Out1 : Outport  Orientation=left
  wires:
  Sum3/1 -> Abs/1, Product/1
  T-/1 -> Sum3/1
  T+/1 -> Sum3/2
  Abs/1 -> Math Function/1
  Constant3/1 -> Math Function/2
  Math Function/1 -> Proportional2/1
  Product/1 -> Out1/1
  Proportional2/1 -> Product/2

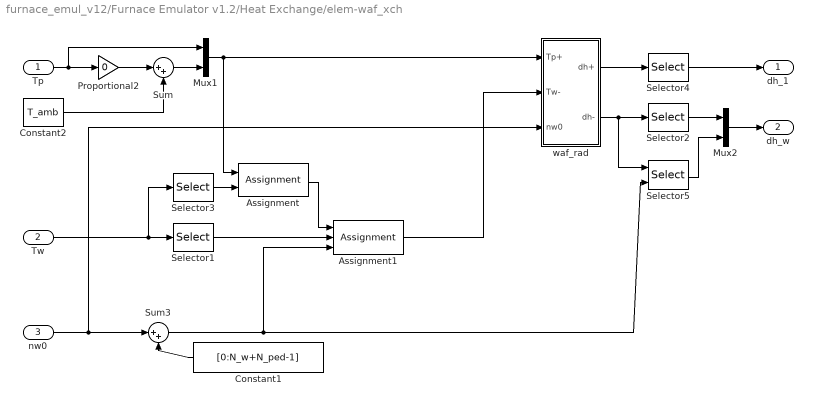
== system furnace_emul_v12/Furnace Emulator v1.2/Heat Exchange/elem-waf_xch ==
  Tp : Inport
  Tw : Inport  Port=2
  nw0 : Inport  Port=3
  Assignment : Assignment  Elements=[1:N_top]
  Assignment1 : Assignment  ElementSrc=External
  Constant1 : Constant  Orientation=left  Value=[0:N_w+N_ped-1]
  Constant2 : Constant  Value=T_amb
  Mux1 : Mux  Inputs=2
  Mux2 : Mux  Inputs=2
  Proportional2 : Gain  Gain=0  SaturateOnIntegerOverflow=on
  Selector1 : Selector  Elements=[N_top+1:N_w+N_ped+N_top]  InputPortWidth=N_w+N_ped+N_top
  Selector2 : Selector  Elements=[1:N_top]  InputPortWidth=2*n
  Selector3 : Selector  Elements=[1:N_top]  InputPortWidth=N_w+N_ped+N_top
  Selector4 : Selector  Elements=[1:n]  InputPortWidth=2*n
  Selector5 : Selector  ElementSrc=External  Elements=[1]  InputPortWidth=2*n
  Sum : Sum  Inputs=|++  SaturateOnIntegerOverflow=on  InputSameDT=on
  Sum3 : Sum  Inputs=|++  SaturateOnIntegerOverflow=on  InputSameDT=on
  waf_rad : Subsystem
  dh_1 : Outport
  dh_w : Outport  Port=2
  wires:
  Mux2/1 -> dh_w/1
  Selector5/1 -> Mux2/2
  Selector2/1 -> Mux2/1
  waf_rad/2(dh-) -> Selector5/1, Selector2/1
  Selector4/1 -> dh_1/1
  waf_rad/1(dh+) -> Selector4/1
  Assignment1/1 -> waf_rad/2(Tw-)
  Sum3/1 -> Selector5/2, Assignment1/3
  Assignment/1 -> Assignment1/1
  Selector1/1 -> Assignment1/2
  Mux1/1 -> waf_rad/1(Tp+), Assignment/1
  Selector3/1 -> Assignment/2
  Constant1/1 -> Sum3/2
  nw0/1 -> waf_rad/3(nw0), Sum3/1
  Tp/1 -> Proportional2/1, Mux1/1
  Proportional2/1 -> Sum/1
  Constant2/1 -> Sum/2
  Tw/1 -> Selector1/1, Selector3/1
  Sum/1 -> Mux1/2

== system furnace_emul_v12/Furnace Emulator v1.2/Heat Exchange/elem_prof_rad ==
  T+ : Inport  Orientation=left
  T- : Inport  Orientation=left  Port=2
  Constant1 : Constant  Value=ones(1,n)  VectorParams1D=off
  Constant2 : Constant  Value=ones(n,1)  VectorParams1D=off
  Constant3 : Constant  Value=F_A_pe
  Product : Product  SaturateOnIntegerOverflow=on  InputSameDT=on
  Product{1..4} (4 alike) : Product  Multiplication=Matrix(*)  SaturateOnIntegerOverflow=on  InputSameDT=on
  Reshape : simulink3/Signals & Systems/Reshape  OutputDimensionality=Column vector  OutputDimensions=[N,N_w]
  Reshape1 : simulink3/Signals & Systems/Reshape  OutputDimensionality=Row vector  OutputDimensions=[N,N_w]
  Reshape2 : simulink3/Signals & Systems/Reshape  OutputDimensionality=1-D array  OutputDimensions=[N,N_w]
  Reshape3 : simulink3/Signals & Systems/Reshape  OutputDimensionality=1-D array  OutputDimensions=[N,N_w]
  elem_prof_rad : Subsystem
  dh+ : Outport  Orientation=left
  dh- : Outport  Orientation=left  Port=2
  wires:
  Constant1/1 -> Product1/2, Product4/1
  Reshape/1 -> Product1/1
  Constant2/1 -> Product2/1, Product3/2
  Reshape1/1 -> Product2/2
  Product1/1 -> elem_prof_rad/1(T+)
  Product2/1 -> elem_prof_rad/2(T-)
  Constant3/1 -> Product/1
  elem_prof_rad/1(DTH) -> Product/2
  Product/1 -> Product3/1, Product4/2
  Product3/1 -> Reshape2/1
  Product4/1 -> Reshape3/1
  T+/1 -> Reshape/1
  T-/1 -> Reshape1/1
  Reshape3/1 -> dh-/1
  Reshape2/1 -> dh+/1

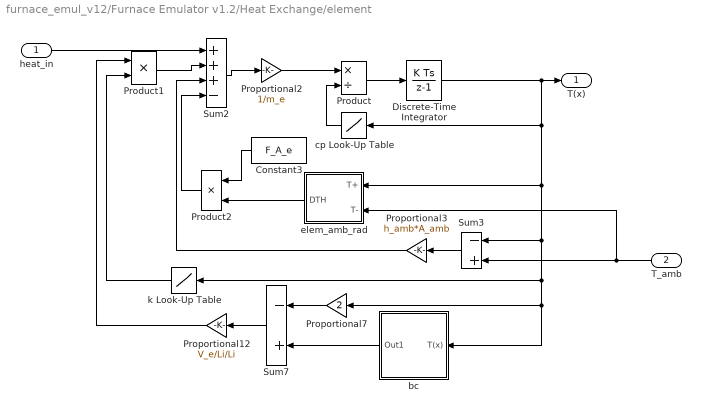
== system furnace_emul_v12/Furnace Emulator v1.2/Heat Exchange/element ==
  heat_in : Inport
  T_amb : Inport  Orientation=left  Port=2
  Constant3 : Constant  Orientation=left  Value=F_A_e
  Discrete-Time Integrator : DiscreteIntegrator  InitialCondition=T_0  SampleTime=Tsa
  Product : Product  Inputs=*/  SaturateOnIntegerOverflow=on  InputSameDT=on
  Product1 : Product  SaturateOnIntegerOverflow=on  InputSameDT=on
  Product2 : Product  Orientation=left  SaturateOnIntegerOverflow=on  InputSameDT=on
  Proportional12 : Gain  Orientation=left  Gain=V_e/Li/Li  SaturateOnIntegerOverflow=on
  Proportional2 : Gain  Gain=1/m_e  SaturateOnIntegerOverflow=on
  Proportional3 : Gain  Orientation=left  Gain=h_amb*A_amb  SaturateOnIntegerOverflow=on
  Proportional7 : Gain  Orientation=left  Gain=2  SaturateOnIntegerOverflow=on
  Sum2 : Sum  Inputs=+++-  SaturateOnIntegerOverflow=on  InputSameDT=on
  Sum3 : Sum  Orientation=left  Inputs=-+  SaturateOnIntegerOverflow=on  InputSameDT=on
  Sum7 : Sum  Orientation=left  Inputs=-+  SaturateOnIntegerOverflow=on  InputSameDT=on
  bc : Subsystem  Orientation=left
  cp Look-Up Table : Lookup  Orientation=left  InputValues=[300,1000]-273  OutputValues=[420, 545]  SaturateOnIntegerOverflow=on
  elem_amb_rad : Subsystem  Orientation=left
  k Look-Up Table : Lookup  Orientation=left  InputValues=[300,1000]-273  OutputValues=[10.8, 21]  SaturateOnIntegerOverflow=on
  T(x) : Outport
  wires:
  heat_in/1 -> Sum2/1
  Sum7/1 -> Proportional12/1
  bc/1(Out1) -> Sum7/2
  Proportional7/1 -> Sum7/1
  T_amb/1 -> Sum3/2, elem_amb_rad/2(T-)
  Discrete-Time Integrator/1 -> T(x)/1, cp Look-Up Table/1, Proportional7/1, bc/1(T(x)), k Look-Up Table/1, Sum3/1, elem_amb_rad/1(T+)
  Sum2/1 -> Proportional2/1
  Proportional12/1 -> Product1/1
  Product/1 -> Discrete-Time Integrator/1
  Proportional2/1 -> Product/1
  cp Look-Up Table/1 -> Product/2
  Product1/1 -> Sum2/2
  k Look-Up Table/1 -> Product1/2
  Sum3/1 -> Proportional3/1
  Proportional3/1 -> Sum2/3
  Product2/1 -> Sum2/4
  elem_amb_rad/1(DTH) -> Product2/2
  Constant3/1 -> Product2/1

== system furnace_emul_v12/Furnace Emulator v1.2/Heat Exchange/gas ==
  Dh_in : Inport
  gas flow : Inport  Port=2
  bc_0 : Inport  Orientation=left  Port=3
  Discrete-Time Integrator : DiscreteIntegrator  InitialCondition=T_a0  SampleTime=Tsa
  Mux : Mux  Orientation=left  Inputs=2
  Product : Product  Inputs=4  SaturateOnIntegerOverflow=on  InputSameDT=on
  Product2 : Product  Inputs=*//  SaturateOnIntegerOverflow=on  InputSameDT=on
  Proportional1 : Gain  Gain=1/V_a  SaturateOnIntegerOverflow=on
  Selector : Selector  Orientation=left  Elements=[1:n-1]  InputPortWidth=n
  Sum1 : Sum  Inputs=+-  SaturateOnIntegerOverflow=on  InputSameDT=on
  Sum5 : Sum  Orientation=left  Inputs=+-  SaturateOnIntegerOverflow=on  InputSameDT=on
  cp Look-Up Table2 : Lookup  Orientation=left  InputValues=[300 500 700 900 1100 1300]-273  OutputValues=[1007 1030 1075 1121 1159 1189]  SaturateOnIntegerOverflow=on
  rho Look-Up Table1 : Lookup  Orientation=left  InputValues=[300 500 700 900 1100 1300 1800]-273  OutputValues=[1.16 0.696 0.496 0.387 0.317 0.286 0.25]  SaturateOnIntegerOverflow=on
  T(x) : Outport
  wires:
  Mux/1 -> Sum5/2
  Selector/1 -> Mux/2
  Sum1/1 -> Proportional1/1
  Discrete-Time Integrator/1 -> rho Look-Up Table1/1, cp Look-Up Table2/1, Sum5/1, Selector/1, T(x)/1
  Sum5/1 -> Product/2
  Dh_in/1 -> Sum1/1
  gas flow/1 -> Product/1
  bc_0/1 -> Mux/1
  rho Look-Up Table1/1 -> Product/4, Product2/2
  cp Look-Up Table2/1 -> Product/3, Product2/3
  Product2/1 -> Discrete-Time Integrator/1
  Proportional1/1 -> Product2/1
  Product/1 -> Sum1/2

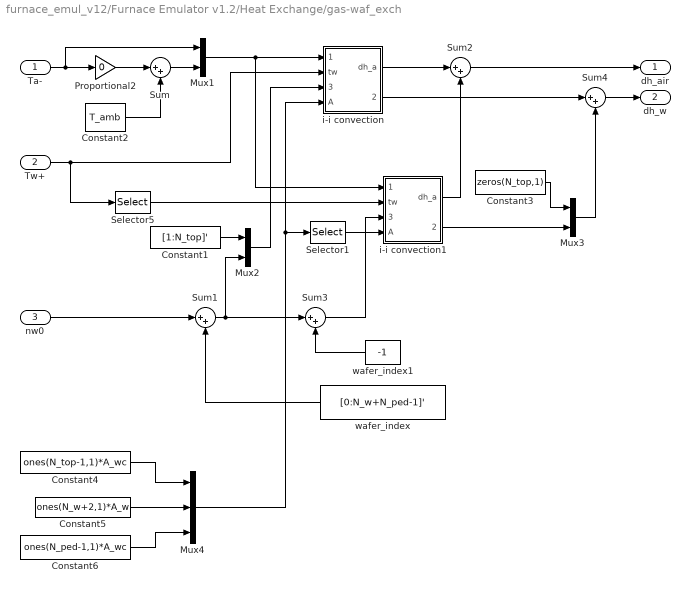
== system furnace_emul_v12/Furnace Emulator v1.2/Heat Exchange/gas-waf_exch ==
  Ta- : Inport
  Tw+ : Inport  Port=2
  nw0 : Inport  Port=3
  Constant1 : Constant  Value=[1:N_top]'
  Constant2 : Constant  Value=T_amb
  Constant3 : Constant  Value=zeros(N_top,1)
  Constant4 : Constant  Value=ones(N_top-1,1)*A_wc
  Constant5 : Constant  Value=ones(N_w+2,1)*A_w
  Constant6 : Constant  Value=ones(N_ped-1,1)*A_wc
  Mux1 : Mux  Inputs=2
  Mux2 : Mux  Inputs=2
  Mux3 : Mux  Inputs=2
  Mux4 : Mux  Inputs=3
  Proportional2 : Gain  Gain=0  SaturateOnIntegerOverflow=on
  Selector1 : Selector  Elements=[1+N_top:N_w+N_ped+N_top]  InputPortWidth=N_w+N_ped+N_top
  Selector5 : Selector  Elements=[1+N_top:N_w+N_ped+N_top]  InputPortWidth=N_w+N_ped+N_top
  Sum{,1..4} (5 alike) : Sum  Inputs=|++  SaturateOnIntegerOverflow=on  InputSameDT=on
  i-i convection : Subsystem
  i-i convection1 : Subsystem
  wafer_index : Constant  Orientation=left  Value=[0:N_w+N_ped-1]'
  wafer_index1 : Constant  Orientation=left  Value=-1
  dh_air : Outport
  dh_w : Outport  Port=2
  wires:
  Ta-/1 -> Proportional2/1, Mux1/1
  Proportional2/1 -> Sum/1
  Constant2/1 -> Sum/2
  Tw+/1 -> Selector5/1, i-i convection/2(tw)
  nw0/1 -> Sum1/1
  wafer_index/1 -> Sum1/2
  Sum/1 -> Mux1/2
  Mux1/1 -> i-i convection/1(ta_t0), i-i convection1/1(ta_t0)
  Sum1/1 -> Sum3/1, Mux2/2
  i-i convection/1(dh_a) -> Sum2/1
  Sum2/1 -> dh_air/1
  wafer_index1/1 -> Sum3/2
  i-i convection1/1(dh_a) -> Sum2/2
  i-i convection/2(dh_w) -> Sum4/1
  Constant1/1 -> Mux2/1
  Mux2/1 -> i-i convection/3(Index)
  Sum3/1 -> i-i convection1/3(Index)
  Mux3/1 -> Sum4/2
  i-i convection1/2(dh_w) -> Mux3/2
  Constant3/1 -> Mux3/1
  Sum4/1 -> dh_w/1
  Selector5/1 -> i-i convection1/2(tw)
  Constant4/1 -> Mux4/1
  Constant5/1 -> Mux4/2
  Constant6/1 -> Mux4/3
  Mux4/1 -> i-i convection/4(A), Selector1/1
  Selector1/1 -> i-i convection1/4(A)

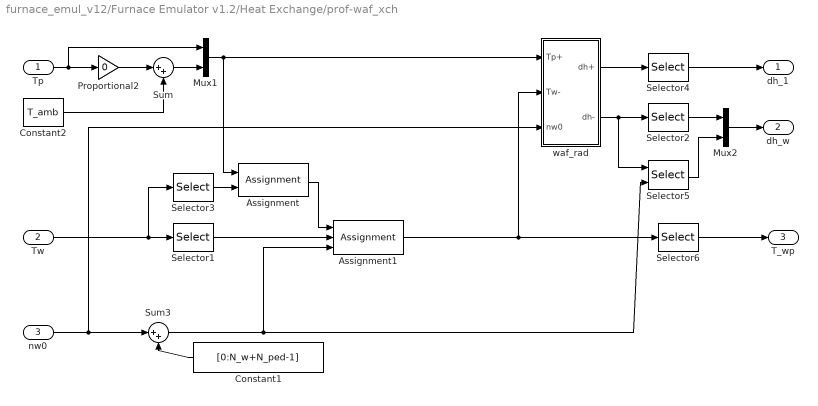
== system furnace_emul_v12/Furnace Emulator v1.2/Heat Exchange/prof-waf_xch ==
  Tp : Inport
  Tw : Inport  Port=2
  nw0 : Inport  Port=3
  Assignment : Assignment  Elements=[1:N_top]
  Assignment1 : Assignment  ElementSrc=External
  Constant1 : Constant  Orientation=left  Value=[0:N_w+N_ped-1]
  Constant2 : Constant  Value=T_amb
  Mux1 : Mux  Inputs=2
  Mux2 : Mux  Inputs=2
  Proportional2 : Gain  Gain=0  SaturateOnIntegerOverflow=on
  Selector1 : Selector  Elements=[N_top+1:N_w+N_ped+N_top]  InputPortWidth=N_w+N_ped+N_top
  Selector2 : Selector  Elements=[1:N_top]  InputPortWidth=2*n
  Selector3 : Selector  Elements=[1:N_top]  InputPortWidth=N_w+N_ped+N_top
  Selector4 : Selector  Elements=[1:n]  InputPortWidth=2*n
  Selector5 : Selector  ElementSrc=External  Elements=[1]  InputPortWidth=2*n
  Selector6 : Selector  Elements=[1:n]  InputPortWidth=2*n
  Sum : Sum  Inputs=|++  SaturateOnIntegerOverflow=on  InputSameDT=on
  Sum3 : Sum  Inputs=|++  SaturateOnIntegerOverflow=on  InputSameDT=on
  waf_rad : Subsystem
  dh_1 : Outport
  dh_w : Outport  Port=2
  T_wp : Outport  Port=3
  wires:
  Sum/1 -> Mux1/2
  Tw/1 -> Selector3/1, Selector1/1
  Constant2/1 -> Sum/2
  Proportional2/1 -> Sum/1
  Tp/1 -> Mux1/1, Proportional2/1
  nw0/1 -> Sum3/1, waf_rad/3(nw0)
  Constant1/1 -> Sum3/2
  Selector3/1 -> Assignment/2
  Mux1/1 -> Assignment/1, waf_rad/1(Tp+)
  Selector1/1 -> Assignment1/2
  Assignment/1 -> Assignment1/1
  Sum3/1 -> Assignment1/3, Selector5/2
  Assignment1/1 -> waf_rad/2(Tw-), Selector6/1
  waf_rad/1(dh+) -> Selector4/1
  Selector4/1 -> dh_1/1
  waf_rad/2(dh-) -> Selector2/1, Selector5/1
  Selector2/1 -> Mux2/1
  Selector5/1 -> Mux2/2
  Mux2/1 -> dh_w/1
  Selector6/1 -> T_wp/1

== system furnace_emul_v12/Furnace Emulator v1.2/Heat Exchange/profile ==
  heat_in : Inport
  T_amb : Inport  Orientation=left  Port=2
  Constant3 : Constant  Orientation=left  Value=F_A_p
  Discrete-Time Integrator : DiscreteIntegrator  InitialCondition=T_0  SampleTime=Tsa
  Product : Product  Inputs=*/  SaturateOnIntegerOverflow=on  InputSameDT=on
  Product1 : Product  SaturateOnIntegerOverflow=on  InputSameDT=on
  Product2 : Product  Orientation=left  SaturateOnIntegerOverflow=on  InputSameDT=on
  Proportional12 : Gain  Orientation=left  Gain=V_p/Li/Li  SaturateOnIntegerOverflow=on
  Proportional2 : Gain  Gain=1/m_p  SaturateOnIntegerOverflow=on
  Proportional7 : Gain  Orientation=left  Gain=2  SaturateOnIntegerOverflow=on
  Selector1 : Selector  Orientation=left  Elements=[1,n]  InputPortWidth=n
  Sum2 : Sum  Inputs=++-  SaturateOnIntegerOverflow=on  InputSameDT=on
  Sum7 : Sum  Orientation=left  Inputs=-+  SaturateOnIntegerOverflow=on  InputSameDT=on
  amb_prof_rad : Subsystem  Orientation=left
  bc : Subsystem  Orientation=left
  cp Look-Up Table1 : Lookup  Orientation=left  InputValues=[400, 600, 800, 1300]-273  OutputValues="[885  1075  1250  1500]"  SaturateOnIntegerOverflow=on
  k Look-Up Table : Lookup  Orientation=left  InputValues=[400, 600, 800, 1300]-273  OutputValues="[7.6  5  4.2  3.2 ]"  SaturateOnIntegerOverflow=on
  T(x) : Outport
  wires:
  Proportional12/1 -> Product1/1
  Sum2/1 -> Proportional2/1
  Discrete-Time Integrator/1 -> T(x)/1, cp Look-Up Table1/1, Proportional7/1, bc/1(T(x)), k Look-Up Table/1, amb_prof_rad/1(T+)
  T_amb/1 -> bc/2(T_amb1,n), amb_prof_rad/2(T-)
  Proportional7/1 -> Sum7/1
  bc/1(Out1) -> Sum7/2
  Sum7/1 -> Proportional12/1
  heat_in/1 -> Sum2/1
  Selector1/1 -> bc/3(K1,n)
  Product1/1 -> Sum2/2
  k Look-Up Table/1 -> Product1/2, Selector1/1
  Proportional2/1 -> Product/1
  Product/1 -> Discrete-Time Integrator/1
  cp Look-Up Table1/1 -> Product/2
  Product2/1 -> Sum2/3
  Constant3/1 -> Product2/1
  amb_prof_rad/1(DTH) -> Product2/2

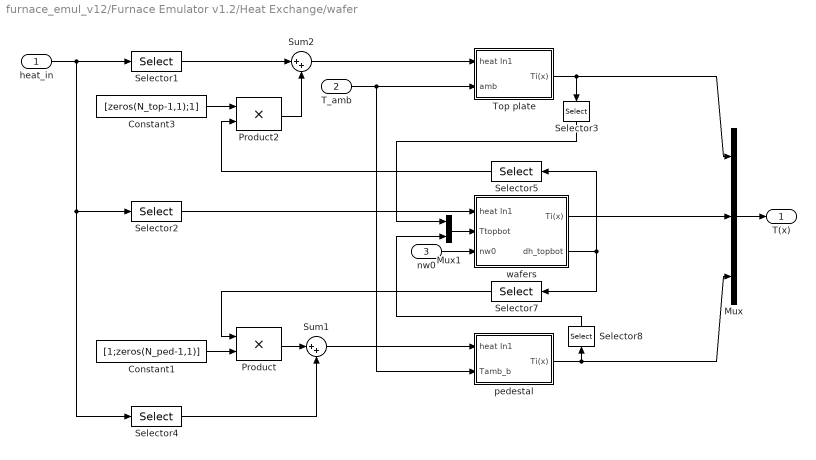
== system furnace_emul_v12/Furnace Emulator v1.2/Heat Exchange/wafer ==
  heat_in : Inport
  T_amb : Inport  Port=2
  nw0 : Inport  Port=3
  Constant1 : Constant  Value=[1;zeros(N_ped-1,1)]
  Constant3 : Constant  Value=[zeros(N_top-1,1);1]
  Mux : Mux  Inputs=3
  Mux1 : Mux  Inputs=2
  Product : Product  SaturateOnIntegerOverflow=on  InputSameDT=on
  Product2 : Product  SaturateOnIntegerOverflow=on  InputSameDT=on
  Selector1 : Selector  Elements=[1:N_top]  InputPortWidth=N_w+N_top+N_ped
  Selector2 : Selector  Elements=[N_top+1:N_w+N_top]  InputPortWidth=N_w+N_top+N_ped
  Selector3 : Selector  Orientation=down  Elements=[N_top]  InputPortWidth=N_top
  Selector4 : Selector  Elements=[N_w+N_top+1:N_w+N_top+N_ped]  InputPortWidth=N_w+N_top+N_ped
  Selector5 : Selector  Orientation=left  InputPortWidth=2
  Selector7 : Selector  Orientation=left  Elements=2  InputPortWidth=2
  Selector8 : Selector  Orientation=up  Elements=[1]  InputPortWidth=N_ped
  Sum1 : Sum  Inputs=|++  SaturateOnIntegerOverflow=on  InputSameDT=on
  Sum2 : Sum  Inputs=|++  SaturateOnIntegerOverflow=on  InputSameDT=on
  Top plate : Subsystem
  pedestal : Subsystem
  wafers : Subsystem
  T(x) : Outport
  wires:
  heat_in/1 -> Selector1/1, Selector2/1, Selector4/1
  Selector1/1 -> Sum2/1
  Selector2/1 -> wafers/1(heat In1)
  Constant1/1 -> Product/2
  Sum1/1 -> pedestal/1(heat In1)
  Top plate/1(Ti(x)) -> Mux/1, Selector3/1
  wafers/1(Ti(x)) -> Mux/2
  pedestal/1(Ti(x)) -> Selector8/1, Mux/3
  Mux/1 -> T(x)/1
  wafers/2(dh_topbot) -> Selector5/1, Selector7/1
  T_amb/1 -> Top plate/2(amb), pedestal/2(Tamb_b)
  Sum2/1 -> Top plate/1(heat In1)
  Mux1/1 -> wafers/2(Ttopbot)
  Selector4/1 -> Sum1/2
  Product/1 -> Sum1/1
  Selector7/1 -> Product/1
  nw0/1 -> wafers/3(nw0)
  Selector8/1 -> Mux1/2
  Product2/1 -> Sum2/2
  Constant3/1 -> Product2/1
  Selector5/1 -> Product2/2
  Selector3/1 -> Mux1/1

== system furnace_emul_v12/Furnace Emulator v1.2/Heat Exchange/elem-waf_xch/waf_rad ==
  Tp+ : Inport  Orientation=left
  Tw- : Inport  Orientation=left  Port=2
  nw0 : Inport  Port=3
  Constant1 : Constant  Value=ones(1,2*n)  VectorParams1D=off
  Constant2 : Constant  Value=ones(2*n,1)  VectorParams1D=off
  MATLAB Fcn : MATLABFcn  MATLABFcn=s_tubew(u,n,N_w,N_ped,F_A_ew,Fb_A_ew,Fs_e)  OutputDimensions=[2*n,2*n]  Output1D=off
  Product : Product  SaturateOnIntegerOverflow=on  InputSameDT=on
  Product{1..4} (4 alike) : Product  Multiplication=Matrix(*)  SaturateOnIntegerOverflow=on  InputSameDT=on
  Reshape : simulink3/Signals & Systems/Reshape  OutputDimensionality=Column vector  OutputDimensions=[N,N_w]
  Reshape1 : simulink3/Signals & Systems/Reshape  OutputDimensionality=Row vector  OutputDimensions=[N,N_w]
  Reshape2 : simulink3/Signals & Systems/Reshape  OutputDimensionality=1-D array  OutputDimensions=[N,N_w]
  Reshape3 : simulink3/Signals & Systems/Reshape  OutputDimensionality=1-D array  OutputDimensions=[N,N_w]
  elem_prof_rad : Subsystem
  dh+ : Outport  Orientation=left
  dh- : Outport  Orientation=left  Port=2
  wires:
  Reshape2/1 -> dh+/1
  Reshape3/1 -> dh-/1
  Tw-/1 -> Reshape1/1
  Tp+/1 -> Reshape/1
  Product4/1 -> Reshape3/1
  Product3/1 -> Reshape2/1
  Product/1 -> Product4/2, Product3/1
  elem_prof_rad/1(DTH) -> Product/2
  MATLAB Fcn/1 -> Product/1
  Product2/1 -> elem_prof_rad/2(T-)
  Product1/1 -> elem_prof_rad/1(T+)
  Reshape1/1 -> Product2/2
  Constant2/1 -> Product2/1, Product3/2
  Reshape/1 -> Product1/1
  Constant1/1 -> Product4/1, Product1/2
  nw0/1 -> MATLAB Fcn/1

== system furnace_emul_v12/Furnace Emulator v1.2/Heat Exchange/elem_prof_rad/elem_prof_rad ==
  T+ : Inport
  T- : Inport  Port=2
  Constant1 : Constant  Value=4
  Constant2 : Constant  Value=273
  Constant3 : Constant  Value=4
  Constant4 : Constant  Value=273
  Math Function : Math  Operator=pow
  Math Function1 : Math  Operator=pow
  Proportional1 : Gain  Gain=5.675  SaturateOnIntegerOverflow=on
  Proportional3 : Gain  Gain=0.01  SaturateOnIntegerOverflow=on
  Proportional4 : Gain  Gain=0.01  SaturateOnIntegerOverflow=on
  Sum1 : Sum  Inputs=2  SaturateOnIntegerOverflow=on  InputSameDT=on
  Sum2 : Sum  Inputs=2  SaturateOnIntegerOverflow=on  InputSameDT=on
  Sum3 : Sum  Inputs=+-  SaturateOnIntegerOverflow=on  InputSameDT=on
  DTH : Outport
  wires:
  Sum3/1 -> Proportional1/1
  Proportional1/1 -> DTH/1
  Math Function1/1 -> Sum3/2
  Math Function/1 -> Sum3/1
  T-/1 -> Sum1/1
  Constant4/1 -> Sum1/2
  Sum1/1 -> Proportional4/1
  Proportional4/1 -> Math Function1/1
  Constant3/1 -> Math Function1/2
  T+/1 -> Sum2/1
  Constant2/1 -> Sum2/2
  Sum2/1 -> Proportional3/1
  Proportional3/1 -> Math Function/1
  Constant1/1 -> Math Function/2

== system furnace_emul_v12/Furnace Emulator v1.2/Heat Exchange/element/bc ==
  T(x) : Inport  Orientation=left
  Mux1 : Mux  Orientation=left  Inputs=2
  Mux2 : Mux  Orientation=left  Inputs=2
  Selector1 : Selector  Orientation=left  Elements=[1:n-1]  InputPortWidth=n
  Selector2 : Selector  Orientation=left  Elements=[2:n]  InputPortWidth=n
  Sum3 : Sum  Orientation=left  Inputs=2  SaturateOnIntegerOverflow=on  InputSameDT=on
  end-point 3 : Fcn  Orientation=left  Expr=u[n]
  end-point 4 : Fcn  Orientation=left  Expr=u[1]
  Out1 : Outport  Orientation=left
  wires:
  end-point 4/1 -> Mux1/1
  end-point 3/1 -> Mux2/2
  Sum3/1 -> Out1/1
  Mux2/1 -> Sum3/1
  Mux1/1 -> Sum3/2
  T(x)/1 -> Selector1/1, end-point 4/1, end-point 3/1, Selector2/1
  Selector1/1 -> Mux1/2
  Selector2/1 -> Mux2/1

== system furnace_emul_v12/Furnace Emulator v1.2/Heat Exchange/element/elem_amb_rad ==
  T+ : Inport
  T- : Inport  Port=2
  Constant1 : Constant  Value=4
  Constant2 : Constant  Value=273
  Constant3 : Constant  Value=4
  Constant4 : Constant  Value=273
  Math Function : Math  Operator=pow
  Math Function1 : Math  Operator=pow
  Proportional1 : Gain  Gain=5.675  SaturateOnIntegerOverflow=on
  Proportional3 : Gain  Gain=0.01  SaturateOnIntegerOverflow=on
  Proportional4 : Gain  Gain=0.01  SaturateOnIntegerOverflow=on
  Sum1 : Sum  Inputs=2  SaturateOnIntegerOverflow=on  InputSameDT=on
  Sum2 : Sum  Inputs=2  SaturateOnIntegerOverflow=on  InputSameDT=on
  Sum3 : Sum  Inputs=+-  SaturateOnIntegerOverflow=on  InputSameDT=on
  DTH : Outport
  wires:
  Constant1/1 -> Math Function/2
  Proportional3/1 -> Math Function/1
  Sum2/1 -> Proportional3/1
  Constant2/1 -> Sum2/2
  T+/1 -> Sum2/1
  Constant3/1 -> Math Function1/2
  Proportional4/1 -> Math Function1/1
  Sum1/1 -> Proportional4/1
  Constant4/1 -> Sum1/2
  T-/1 -> Sum1/1
  Math Function/1 -> Sum3/1
  Math Function1/1 -> Sum3/2
  Proportional1/1 -> DTH/1
  Sum3/1 -> Proportional1/1
